simulink model "GS_model"  (R2018b)
settings: Solver=ode5  StartTime=0.0  StopTime=SimuStopTime  FixedStep=T_Simu  RelTol=1e-3
InitFcn:
  | Initial
undefined symbols (not defined in the file or in its folder): Aba10, Aba20, aeroCIP2006_S, aeroCIP2006_X, aeroCIP2006_Y, Agl0, Ass_kS, Ass_n1, Ass_n2, Ass_n3, Ass_n4, Ass_Noise, Ass_R, Ass_Resolution, Ass_TmOrder, AssA_Fix_Abs, AssB_Fix_Abs, AssC_Fix_Abs, AssD_Fix_Abs, AssE_Fix_Aps, AssF_Fix_Aps, C, c_max, c_min, Cd, CenterOfFigNX, CenterOfFigNY, CenterOfFigNZ, CenterOfFigP1, CenterOfFigP2, CenterOfFigPX, CenterOfFigPY, CenterOfFigPZ, Cmu, Crou, DEG2RAD, DiscIntNeverNeededParam, Eg_Dir, Eg_F, Eg_PrepareTime, Eg_r_L_L, Fw_Abf, Fw_Hmax, Fw_J, Fw_Spd0, Fw_Tmax, git_hash_BaseLine, git_hash_Project, Gnss_Noise_Pos, Gnss_Noise_Vel, Gnss_PropgationTime, GyroA_Fix_Abg, GyroA_Noise, GyroB_Fix_Abg, GyroB_Noise, GyroC_Fix_Abg, GyroC_Noise, GyroD_Fix_Abg, GyroD_Noise, h ... (+94)
libraries: simulink x308, sharedutil x46, aerolibutil x37, sharedtransform x31, vrlib x14, aerolibgravity2 x2
(part 5 of 20)

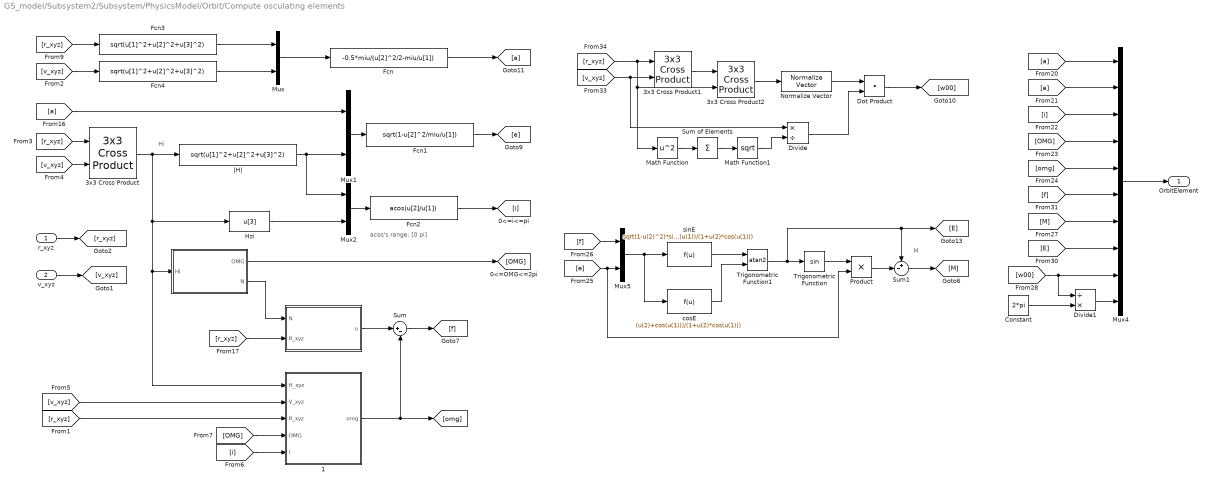
== system GS_model/Subsystem2/Subsystem/PhysicsModel/Orbit/Compute osculating elements ==
  note: Hi
  note: acos's range: [0 pi]
  note: M
  r_xyz : Inport
  v_xyz : Inport  Port=2
  " " : Subsystem
  "     " : Subsystem
  "   1" : Subsystem
  3x3 Cross Product : sharedutil/3x3 Cross Product  aMode=aMode
      settings: SourceProductBaseCode=AE,PW,MT,VE,VP
  3x3 Cross Product1 : sharedutil/3x3 Cross Product  aMode=aMode
      settings: SourceProductBaseCode=AE,PW,MT,VE,VP
  3x3 Cross Product2 : sharedutil/3x3 Cross Product  aMode=aMode
      settings: SourceProductBaseCode=AE,PW,MT,VE,VP
  Constant : Constant  Value=2*pi
  Divide : Product  Inputs=*/
  Divide1 : Product  Inputs=/*
  Dot Product : DotProduct  InputSameDT=on  OutDataTypeStr=Inherit: Inherit via internal rule
  Fcn : Fcn  Expr=-0.5*miu/(u[2]^2/2-miu/u[1])
  Fcn1 : Fcn  Expr=sqrt(1-u[2]^2/miu/u[1])
  Fcn2 : Fcn  Expr=acos(u[2]/u[1])
  Fcn3 : Fcn  Expr=sqrt(u[1]^2+u[2]^2+u[3]^2)
  Fcn4 : Fcn  Expr=sqrt(u[1]^2+u[2]^2+u[3]^2)
  Hzi : Fcn  Expr=u[3]
  Math Function : Math  Operator=square  SaturateOnIntegerOverflow=on
  Math Function1 : Math  Operator=sqrt  SaturateOnIntegerOverflow=on
  Mux{,1..2,5} (4 alike) : Mux  Inputs=2
  Mux4 : Mux  Inputs=10
  Normalize Vector : vrlib/Utilities/Normalize Vector  maxzero=0
  Product : Product  RndMeth=Zero
  Sum : Sum  Inputs=|+-
  Sum of Elements : Sum  Inputs=+
  Sum1 : Sum  Inputs=+-|
  Trigonometric Function : Trigonometry
  Trigonometric Function1 : Trigonometry  Operator=atan2
  cosE : Fcn  Expr=(u(2)+cos(u(1)))/(1+u(2)*cos(u(1)))
  sinE : Fcn  Expr=sqrt(1-u(2)^2)*sin(u(1))/(1+u(2)*cos(u(1)))
  |H| : Fcn  Expr=sqrt(u[1]^2+u[2]^2+u[3]^2)
  OrbitElement : Outport
  wires:
  [r_xyz] -> Fcn3/1
  [v_xyz] -> Fcn4/1
  Fcn4/1 -> Mux/2
  Mux/1 -> Fcn/1
  Fcn/1 -> [a]
  3x3 Cross Product/1 -> |H|/1, "   1"/1(H_xyz), " "/1(Hi), Hzi/1
  Mux1/1 -> Fcn1/1
  Mux2/1 -> Fcn2/1
  r_xyz/1 -> [r_xyz]
  v_xyz/1 -> [v_xyz]
  [r_xyz] -> "   1"/3(R_xyz)
  [r_xyz] -> 3x3 Cross Product/1
  [v_xyz] -> 3x3 Cross Product/2
  [v_xyz] -> "   1"/2(V_xyz)
  Fcn3/1 -> Mux/1
  |H|/1 -> Mux1/2, Mux2/1
  " "/1(OMG) -> [OMG]
  Fcn1/1 -> [e]
  Fcn2/1 -> [i]
  [a] -> Mux1/1
  "   1"/1(omg) -> Sum/2, [omg]
  Hzi/1 -> Mux2/2
  "     "/1(u) -> Sum/1
  [r_xyz] -> "     "/2(R_xyz)
  Sum/1 -> [f]
  [f] -> Mux5/1
  [e] -> Mux5/2, Product/2
  Mux5/1 -> sinE/1, cosE/1
  Trigonometric Function/1 -> Product/1
  Product/1 -> Sum1/2
  Sum1/1 -> [M]
  Dot Product/1 -> [w00]
  Mux4/1 -> OrbitElement/1
  sinE/1 -> Trigonometric Function1/1
  cosE/1 -> Trigonometric Function1/2
  Trigonometric Function1/1 -> Sum1/1, [E], Trigonometric Function/1
  [r_xyz] -> 3x3 Cross Product1/1, 3x3 Cross Product2/2, Math Function/1
  [v_xyz] -> 3x3 Cross Product1/2, Divide/1
  3x3 Cross Product1/1 -> 3x3 Cross Product2/1
  3x3 Cross Product2/1 -> Normalize Vector/1
  Normalize Vector/1 -> Dot Product/1
  Sum of Elements/1 -> Math Function1/1
  Math Function/1 -> Sum of Elements/1
  Math Function1/1 -> Divide/2
  Divide/1 -> Dot Product/2
  [a] -> Mux4/1
  [e] -> Mux4/2
  [i] -> Mux4/3
  [OMG] -> Mux4/4
  [omg] -> Mux4/5
  [f] -> Mux4/6
  [M] -> Mux4/7
  [E] -> Mux4/8
  [w00] -> Divide1/1, Mux4/9
  Divide1/1 -> Mux4/10
  Constant/1 -> Divide1/2
  " "/2(N) -> "     "/1(N)
  [i] -> "   1"/5(i)
  [OMG] -> "   1"/4(OMG)

== system GS_model/Subsystem2/Subsystem/PhysicsModel/Orbit/Engine ==
  F_Engine(b) : Inport
  Qib : Inport  Port=2
  Math Function : Math  Operator=transpose  SaturateOnIntegerOverflow=on
  Product2 : Product  Multiplication=Matrix(*)
  Quaternions to Direction Cosine Matrix1 : sharedtransform/Quaternions to  Direction Cosine Matrix  aMode=aMode
      settings: SourceProductBaseCode=AE,PW,MT,VE,VP
  F_Engine(i) : Outport
  wires:
  F_Engine(b)/1 -> Product2/2
  Math Function/1 -> Product2/1
  Product2/1 -> F_Engine(i)/1
  Qib/1 -> Quaternions to Direction Cosine Matrix1/1
  Quaternions to Direction Cosine Matrix1/1 -> Math Function/1

== system GS_model/Subsystem2/Subsystem/PhysicsModel/Orbit/Qob 2 Qib ==
  note: u
  note: i
  note: OMG
  OrbitElement : Inport
  Fcn : Fcn  Expr=u(4)
  Fcn1 : Fcn  Expr=u(3)
  Fcn2 : Fcn  Expr=u(5)+u(6)
  Mux : Mux  Inputs=3
  Quaternion Multiplication : aerolibutil/Quaternion Multiplication
  Rotation Angles to Quaternions : sharedtransform/Rotation Angles to Quaternions  rotationOrder=ZXZ  aMode=aMode
      settings: SourceProductBaseCode=AE,PW,MT,VE,VP
  qpo : Constant  Value=[0.5 -0.5 -0.5 0.5]
  Qio : Outport
  wires:
  Rotation Angles to Quaternions/1 -> Quaternion Multiplication/1
  qpo/1 -> Quaternion Multiplication/2
  Quaternion Multiplication/1 -> Qio/1
  OrbitElement/1 -> Fcn2/1, Fcn/1, Fcn1/1
  Fcn1/1 -> Mux/2
  Fcn/1 -> Mux/1
  Fcn2/1 -> Mux/3
  Mux/1 -> Rotation Angles to Quaternions/1

== system GS_model/Subsystem2/Subsystem/PhysicsModel/Orbit/RV_i2RV_f ==
  R_i : Inport
  V_i : Inport  Port=2
  Afi : Inport  Port=3
  Constant : Constant  Value=[0;0;we]
  Cross Product : vrlib/Utilities/Cross Product
  MatrixMultiply : Product  Multiplication=Matrix(*)
  MatrixMultiply1 : Product  Multiplication=Matrix(*)
  Sum : Sum  Inputs=-+|
  R_f : Outport
  V_f : Outport  Port=2
  wires:
  MatrixMultiply/1 -> Cross Product/2, R_f/1
  Afi/1 -> MatrixMultiply/1, MatrixMultiply1/1
  R_i/1 -> MatrixMultiply/2
  V_i/1 -> MatrixMultiply1/2
  MatrixMultiply1/1 -> Sum/2
  Constant/1 -> Cross Product/1
  Cross Product/1 -> Sum/1
  Sum/1 -> V_f/1

== system GS_model/Subsystem2/Subsystem/PhysicsModel/Orbit/Subsystem ==
  Tc_Orbit_Reset : Inport
  RV0 : Inport  Port=2
  a_Perturbation : Inport  Port=3
  F_EP : Inport  Port=4
  Demux : Demux  Outputs=[3;3]
  Gain : Gain  Gain=1/m
  Integrator : Integrator  ExternalReset=level  InitialConditionSource=external
  Integrator1 : Integrator  ExternalReset=level  InitialConditionSource=external
  Sum : Sum  Inputs=|++
  R_i : Outport
  V_i : Outport  Port=2
  wires:
  Integrator/1 -> Integrator1/1, V_i/1
  Tc_Orbit_Reset/1 -> Integrator1/2, Integrator/2
  F_EP/1 -> Gain/1
  Sum/1 -> Integrator/1
  a_Perturbation/1 -> Sum/1
  Demux/1 -> Integrator1/3
  Demux/2 -> Integrator/3
  Integrator1/1 -> R_i/1
  RV0/1 -> Demux/1
  Gain/1 -> Sum/2

== system GS_model/Subsystem2/Subsystem/PhysicsModel/Orbit/Subsystem1 ==
  UTC_1970 : Inport
  Constant : Constant  Value=aeroCIP2006_X
  Constant1 : Constant  Value=aeroCIP2006_Y
  Constant3 : Constant  Value=aeroCIP2006_S
  DcmECI2ECEF : MATLAB Function  TreatAsAtomicUnit=on
  Demux : Demux  Outputs=14
  From File : FromFile  FileName=EOP_data_in.mat  OutDataTypeStr=double  SampleTime=0
  Gain{3..6} (4 alike) : Gain  Gain=1/3600/180*pi
  Mux : Mux  Inputs=2
  Mux1 : Mux  Inputs=2
  Terminator{,1..7} (8 alike) : Terminator
  Afi : Outport
  wires:
  Demux/7 -> Gain4/1
  Demux/9 -> Terminator4/1
  From File/1 -> Demux/1
  Demux/14 -> DcmECI2ECEF/7(deltaAT)
  Demux/13 -> Gain6/1
  Gain6/1 -> Mux1/2
  Demux/11 -> Terminator6/1
  Mux1/1 -> DcmECI2ECEF/6(dCIP)
  Demux/6 -> Gain3/1
  Demux/4 -> Terminator2/1
  Demux/3 -> Terminator1/1
  Demux/8 -> DcmECI2ECEF/5(deltaUT1)
  Gain5/1 -> Mux1/1
  Demux/5 -> Terminator3/1
  Demux/12 -> Gain5/1
  Mux/1 -> DcmECI2ECEF/4(polarMotion)
  Gain3/1 -> Mux/1
  Gain4/1 -> Mux/2
  Demux/10 -> Terminator5/1
  Demux/2 -> Terminator/1
  Demux/1 -> Terminator7/1
  UTC_1970/1 -> DcmECI2ECEF/8(Seconds)
  DcmECI2ECEF/1(y) -> Afi/1
  Constant/1 -> DcmECI2ECEF/2(aeroCIP2006_X)
  Constant1/1 -> DcmECI2ECEF/1(aeroCIP2006_Y)
  Constant3/1 -> DcmECI2ECEF/3(aeroCIP2006_S)

== system GS_model/Subsystem2/Subsystem/PhysicsModel/Subsystem3/Subsystem1 ==
  note: A_a0a
  note: A_p0p
  Agl/w/a_SADA : Inport
  Constant : Constant  Value=round(SADA_RotateOrder/100)
  Constant1 : Constant  Value=Aba10
  Constant2 : Constant  Value=Aba20
  Constant3 : Constant  Value=round(mod(SADA_RotateOrder,100)/10)
  MATLAB Function : MATLAB Function  TreatAsAtomicUnit=on
  MATLAB Function1 : MATLAB Function  TreatAsAtomicUnit=on
  MATLAB Function2 : MATLAB Function  TreatAsAtomicUnit=on
  MATLAB Function3 : MATLAB Function  TreatAsAtomicUnit=on
  Product{1..4} (4 alike) : Product  Multiplication=Matrix(*)  SaturateOnIntegerOverflow=on  InputSameDT=on  OutDataTypeStr=Inherit: Same as first input
  Selector : Selector  InputPortWidth=12  IndexOptions=Index vector (dialog)  Indices=[1]  OutputSizes=1
  Selector1 : Selector  InputPortWidth=12  IndexOptions=Index vector (dialog)  Indices=7  OutputSizes=1
  Selector4 : Selector  InputPortWidth=12  IndexOptions=Index vector (dialog)  Indices=4  OutputSizes=1
  Selector5 : Selector  InputPortWidth=12  IndexOptions=Index vector (dialog)  Indices=10  OutputSizes=1
  Transpose{,1..3} (4 alike) : Math  Operator=transpose  SaturateOnIntegerOverflow=on
  Abp1 : Outport
  Aba1 : Outport  Port=2
  Abp2 : Outport  Port=3
  Aba2 : Outport  Port=4
  wires:
  Transpose/1 -> Product2/2
  Transpose3/1 -> Product4/2
  Selector/1 -> MATLAB Function/1(Agl)
  Transpose2/1 -> Product3/2
  MATLAB Function3/1(A) -> Transpose3/1
  MATLAB Function/1(A) -> Transpose/1
  Transpose1/1 -> Product1/2
  Constant1/1 -> Product2/1
  Agl/w/a_SADA/1 -> Selector/1, Selector5/1, Selector1/1, Selector4/1
  Constant2/1 -> Product3/1
  MATLAB Function2/1(A) -> Transpose2/1
  MATLAB Function1/1(A) -> Transpose1/1
  Constant/1 -> MATLAB Function2/2(Order), MATLAB Function/2(Order)
  Selector4/1 -> MATLAB Function1/1(Agl)
  Constant3/1 -> MATLAB Function1/2(Order), MATLAB Function3/2(Order)
  Selector1/1 -> MATLAB Function2/1(Agl)
  Selector5/1 -> MATLAB Function3/1(Agl)
  Product2/1 -> Product1/1, Aba1/1
  Product1/1 -> Abp1/1
  Product3/1 -> Product4/1, Aba2/1
  Product4/1 -> Abp2/1

== system GS_model/Subsystem2/Subsystem/PhysicsModel/Time/Subsystem ==
  In1 : Inport
  Trigger : TriggerPort  TriggerType=falling  VariantControl=Variant  PortDimensions=1
  Out1 : Outport
  wires:
  In1/1 -> Out1/1

== system GS_model/Subsystem2/Subsystem/Sensor/Ass/BodyAss(A&B&C&D)Model ==
  Sunshine : Inport
  Sun_b : Inport  Port=2
  TC_Ass : Inport  Port=3
  Constant : Constant  Value=AssA_Fix_Abs
  Constant1 : Constant  Value=Ass_kS
  Constant2 : Constant
  Constant3 : Constant  Value=AssB_Fix_Abs
  Constant4 : Constant  Value=AssC_Fix_Abs
  Constant5 : Constant  Value=AssD_Fix_Abs
  Constant6 : Constant  Value=2
  Constant7 : Constant  Value=3
  Constant8 : Constant  Value=4
  Mux : Mux
  Subsystem : Subsystem
      mask Display: disp('AssAModel')
  Subsystem1 : Subsystem
      mask Display: disp('AssAModel')
  Subsystem2 : Subsystem
      mask Display: disp('AssAModel')
  Subsystem3 : Subsystem
      mask Display: disp('AssAModel')
  TM_Data_AssA&B&C&D : Outport
  wires:
  Subsystem3/1(TM_Data_AssA) -> Mux/4
  Sun_b/1 -> Subsystem1/3(Sun_b), Subsystem3/3(Sun_b), Subsystem2/3(Sun_b), Subsystem/3(Sun_b)
  Sunshine/1 -> Subsystem1/1(Sunshine), Subsystem3/1(Sunshine), Subsystem2/1(Sunshine), Subsystem/1(Sunshine)
  Subsystem1/1(TM_Data_AssA) -> Mux/2
  Constant1/1 -> Subsystem1/4(kS_Ass), Subsystem3/4(kS_Ass), Subsystem2/4(kS_Ass), Subsystem/4(kS_Ass)
  Constant5/1 -> Subsystem3/2(AbAss)
  TC_Ass/1 -> Subsystem1/5(TC_Ass), Subsystem3/5(TC_Ass), Subsystem2/5(TC_Ass), Subsystem/5(TC_Ass)
  Constant/1 -> Subsystem/2(AbAss)
  Constant3/1 -> Subsystem1/2(AbAss)
  Constant4/1 -> Subsystem2/2(AbAss)
  Subsystem/1(TM_Data_AssA) -> Mux/1
  Subsystem2/1(TM_Data_AssA) -> Mux/3
  Mux/1 -> TM_Data_AssA&B&C&D/1
  Constant2/1 -> Subsystem/6(AssNum)
  Constant6/1 -> Subsystem1/6(AssNum)
  Constant7/1 -> Subsystem2/6(AssNum)
  Constant8/1 -> Subsystem3/6(AssNum)

== system GS_model/Subsystem2/Subsystem/Sensor/Ass/SolarPanelAss(E&F)Model ==
  Sunshine : Inport
  Sun_b : Inport  Port=2
  TC_Ass : Inport  Port=3
  Abp_PY : Inport  Port=4
  Abp_NY : Inport  Port=5
  Constant : Constant  Value=AssE_Fix_Aps
  Constant1 : Constant  Value=Ass_kS
  Constant2 : Constant  Value=5
  Constant3 : Constant  Value=AssF_Fix_Aps
  Constant4 : Constant  Value=6
  Mux : Mux  Inputs=2
  Subsystem : Subsystem
      mask Display: disp('AssEModel')
  Subsystem1 : Subsystem
      mask Display: disp('AssFModel')
  TM_Data_AssE&F : Outport
  wires:
  Mux/1 -> TM_Data_AssE&F/1
  Subsystem/1(TM_Data_AssE) -> Mux/1
  Constant3/1 -> Subsystem1/2(ApAss)
  Constant/1 -> Subsystem/2(ApAss)
  Constant1/1 -> Subsystem1/4(kS_Ass), Subsystem/4(kS_Ass)
  Subsystem1/1(TM_Data_AssF) -> Mux/2
  Sunshine/1 -> Subsystem1/1(Sunshine), Subsystem/1(Sunshine)
  Sun_b/1 -> Subsystem1/3(Sun_b), Subsystem/3(Sun_b)
  Abp_PY/1 -> Subsystem/6(Abp_PY)
  TC_Ass/1 -> Subsystem1/5(TC_Ass), Subsystem/5(TC_Ass)
  Abp_NY/1 -> Subsystem1/6(Abp_NY)
  Constant2/1 -> Subsystem/7(AssNum)
  Constant4/1 -> Subsystem1/7(AssNum)

== system GS_model/Subsystem2/Subsystem/Sensor/GNSS/Enabled Subsystem ==
  In1 : Inport
  Trigger : TriggerPort  VariantControl=Variant  PortDimensions=1
  Out1 : Outport
  wires:
  In1/1 -> Out1/1

== system GS_model/Subsystem2/Subsystem/Sensor/GNSS/GNSSErrModel ==
  note: TC_GNSS_GNDSet_Pos[4*1]
  note: TC_GNSSErr_Pos_Constant[2*1]
  note: TC_GNSSErr_Spd_Constant[2*1]
  note: TC_GNSSErr_Pos_WildValue[1*1]
  note: TC_GNSSErr_Spd_WildValue[1*1]
  note: TC_GNSS_GNDSet_Spd[4*1]
  note: TC_GNSS_PropagationTime[1*1]
  TC_GNSS : Inport
  R_84 : Inport  Port=2
  V_84 : Inport  Port=3
  Demux : Demux  Outputs=[4;2;1;4;2;1;2]
  GNSSErrSet_Pos : Subsystem
      mask Display: disp('GNSSErrSet_Constant')
  GNSSErrSet_Pos1 : Subsystem
      mask Display: disp('GNSSErrSet_WildValue')
  TM_R_84 : Outport
  TM_V_84 : Outport  Port=2
  TC_GNSS_PropagationTime : Outport  Port=3
  wires:
  TC_GNSS/1 -> Demux/1
  Demux/6 -> GNSSErrSet_Pos1/3(TC_GNSSErr_Spd_WildValue)
  Demux/5 -> GNSSErrSet_Pos1/2(TC_GNSSErr_Spd_Constant)
  Demux/3 -> GNSSErrSet_Pos/4(TC_GNSSErr_Pos_WildValue)
  Demux/1 -> GNSSErrSet_Pos/2(TC_GNSS_GNDSet_Pos)
  Demux/2 -> GNSSErrSet_Pos/3(TC_GNSSErr_Pos_Constant)
  R_84/1 -> GNSSErrSet_Pos/1(R_84)
  Demux/4 -> GNSSErrSet_Pos1/1(TC_GNSS_GNDSet_Spd)
  V_84/1 -> GNSSErrSet_Pos1/4(V_84)
  GNSSErrSet_Pos/1(TM_R_84) -> TM_R_84/1
  GNSSErrSet_Pos1/1(TM_V_84) -> TM_V_84/1
  Demux/7 -> TC_GNSS_PropagationTime/1

== system GS_model/Subsystem2/Subsystem/Sensor/GNSS/GNSS_IntegerSecond_Judge ==
  TAI1970 : Inport
  Compare To Constant : simulink/Logic and Bit Operations/Compare To Constant  relop=<=  const=T_Simu/2  OutDataTypeStr=boolean
  Compare To Constant1 : simulink/Logic and Bit Operations/Compare To Constant  relop=<  const=T_Simu/2  OutDataTypeStr=boolean
  Constant : Constant
  Logical Operator : Logic  Operator=OR  AllPortsSameDT=off  OutDataTypeStr=boolean
  Math Function : Math  Operator=mod  SaturateOnIntegerOverflow=on
  Sum : Sum  Inputs=|+-
  Boolean : Outport
  wires:
  Sum/1 -> Compare To Constant1/1
  Math Function/1 -> Sum/2, Compare To Constant/1
  Constant/1 -> Math Function/2, Sum/1
  Compare To Constant1/1 -> Logical Operator/1
  Compare To Constant/1 -> Logical Operator/2
  TAI1970/1 -> Math Function/1
  Logical Operator/1 -> Boolean/1

== system GS_model/Subsystem2/Subsystem/Sensor/GNSS/Orbit ==
  note: a
  note: e
  note: i
  note: OMG
  note: omg
  note: M
  note: E
  note: w00
  note: w00/2pi
  note: f0+T*w0
  "\tTC_GNSS_PropagationTime" : Inport
  UTC_1970 : Inport  Port=2
  Demux : Demux  Outputs=2
  Demux1 : Demux  Outputs=10
  Dot Product1 : DotProduct  InputSameDT=on  OutDataTypeStr=Inherit: Inherit via internal rule
  MATLAB Function2 : MATLAB Function  TreatAsAtomicUnit=on
  Mux4 : Mux  Inputs=10
  RV_i2RV_f1 : Subsystem
  Subsystem1 : Subsystem
  Sum : Sum  Inputs=|++
  Sum1 : Sum  Inputs=|++
  R_f : Outport
  V_f : Outport  Port=2
  wires:
  Mux4/1 -> MATLAB Function2/1(Orbit)
  Subsystem1/1(Afi) -> RV_i2RV_f1/3(Afi)
  MATLAB Function2/1(RV_i) -> Demux/1
  Demux/1 -> RV_i2RV_f1/1(R_i)
  Demux/2 -> RV_i2RV_f1/2(V_i)
  RV_i2RV_f1/1(R_f) -> R_f/1
  RV_i2RV_f1/2(V_f) -> V_f/1
  [Orbit] -> Demux1/1
  Demux1/1 -> Mux4/1
  Demux1/2 -> Mux4/2
  Demux1/3 -> Mux4/3
  Demux1/4 -> Mux4/4
  Demux1/5 -> Mux4/5
  Demux1/7 -> Mux4/7
  Demux1/8 -> Mux4/8
  Demux1/9 -> Mux4/9, Dot Product1/1
  Demux1/10 -> Mux4/10
  Sum/1 -> Mux4/6
  "\tTC_GNSS_PropagationTime"/1 -> Sum1/2, Dot Product1/2
  Dot Product1/1 -> Sum/2
  Demux1/6 -> Sum/1
  UTC_1970/1 -> Sum1/1
  Sum1/1 -> Subsystem1/1(UTC_1970)

== system GS_model/Subsystem2/Subsystem/Sensor/GNSS/Orbit1 ==
  note: f0+T*w0
  note: w00/2pi
  note: w00
  note: E
  note: M
  note: omg
  note: OMG
  note: i
  note: e
  note: a
  "\tTC_GNSS_PropagationTime" : Inport
  UTC_1970 : Inport  Port=2
  Demux : Demux  Outputs=2
  Demux1 : Demux  Outputs=10
  Dot Product1 : DotProduct  InputSameDT=on  OutDataTypeStr=Inherit: Inherit via internal rule
  MATLAB Function2 : MATLAB Function  TreatAsAtomicUnit=on
  Mux4 : Mux  Inputs=10
  RV_i2RV_f1 : Subsystem
  Subsystem1 : Subsystem
  Sum : Sum  Inputs=|++
  Sum1 : Sum  Inputs=|++
  R_f : Outport
  V_f : Outport  Port=2
  wires:
  Sum1/1 -> Subsystem1/1(UTC_1970)
  UTC_1970/1 -> Sum1/1
  Demux1/6 -> Sum/1
  Dot Product1/1 -> Sum/2
  "\tTC_GNSS_PropagationTime"/1 -> Dot Product1/2, Sum1/2
  Sum/1 -> Mux4/6
  Demux1/10 -> Mux4/10
  Demux1/9 -> Dot Product1/1, Mux4/9
  Demux1/8 -> Mux4/8
  Demux1/7 -> Mux4/7
  Demux1/5 -> Mux4/5
  Demux1/4 -> Mux4/4
  Demux1/3 -> Mux4/3
  Demux1/2 -> Mux4/2
  Demux1/1 -> Mux4/1
  [Orbit] -> Demux1/1
  RV_i2RV_f1/2(V_f) -> V_f/1
  RV_i2RV_f1/1(R_f) -> R_f/1
  Demux/2 -> RV_i2RV_f1/2(V_i)
  Demux/1 -> RV_i2RV_f1/1(R_i)
  MATLAB Function2/1(RV_i) -> Demux/1
  Subsystem1/1(Afi) -> RV_i2RV_f1/3(Afi)
  Mux4/1 -> MATLAB Function2/1(Orbit)

== system GS_model/Subsystem2/Subsystem/Sensor/Gyro/GyroAModel ==
  Wbi_b : Inport
  Gyro_Fix_Abg : Inport  Port=2
  Gyro_Noise : Inport  Port=3
  TC_Gyro : Inport  Port=4
  Gyro_Num : Inport  Port=5
  Demux : Demux  Outputs=[20;4]
  GyroErrSet : Subsystem
  GyroMathModel : Subsystem
  TM_Gyro_Wgi : Outport
  wires:
  Wbi_b/1 -> GyroMathModel/1(Wbi_b)
  Gyro_Fix_Abg/1 -> GyroMathModel/2(Gyro_Fix_Abg)
  Gyro_Noise/1 -> GyroMathModel/4(Gyro_Noise)
  Gyro_Num/1 -> GyroErrSet/3(Gyro_Num), GyroMathModel/5("Gyro_Num ")
  GyroMathModel/1(Wgi_g) -> GyroErrSet/1(Wgi)
  GyroErrSet/1(TM_Gyro_Wgi) -> TM_Gyro_Wgi/1
  TC_Gyro/1 -> Demux/1
  Demux/1 -> GyroErrSet/2(TC_Gyro)
  Demux/2 -> GyroMathModel/3(Gyro_Drift)

== system GS_model/Subsystem2/Subsystem/Sensor/Gyro/GyroBModel ==
  Wbi_b : Inport
  Gyro_Fix_Abg : Inport  Port=2
  Gyro_Noise : Inport  Port=3
  TC_Gyro : Inport  Port=4
  Gyro_Num : Inport  Port=5
  Demux : Demux  Outputs=[20;4]
  GyroErrSet : Subsystem
  GyroMathModel : Subsystem
  TM_Gyro_Wgi : Outport
  wires:
  Demux/2 -> GyroMathModel/3(Gyro_Drift)
  Demux/1 -> GyroErrSet/2(TC_Gyro)
  TC_Gyro/1 -> Demux/1
  GyroErrSet/1(TM_Gyro_Wgi) -> TM_Gyro_Wgi/1
  GyroMathModel/1(Wgi_g) -> GyroErrSet/1(Wgi)
  Gyro_Num/1 -> GyroErrSet/3(Gyro_Num), GyroMathModel/5("Gyro_Num ")
  Gyro_Noise/1 -> GyroMathModel/4(Gyro_Noise)
  Gyro_Fix_Abg/1 -> GyroMathModel/2(Gyro_Fix_Abg)
  Wbi_b/1 -> GyroMathModel/1(Wbi_b)

== system GS_model/Subsystem2/Subsystem/Sensor/Gyro/GyroCModel ==
  Wbi_b : Inport
  Gyro_Fix_Abg : Inport  Port=2
  Gyro_Noise : Inport  Port=3
  TC_Gyro : Inport  Port=4
  Gyro_Num : Inport  Port=5
  Demux : Demux  Outputs=[20;4]
  GyroErrSet : Subsystem
  GyroMathModel : Subsystem
  TM_Gyro_Wgi : Outport
  wires:
  Wbi_b/1 -> GyroMathModel/1(Wbi_b)
  Gyro_Fix_Abg/1 -> GyroMathModel/2(Gyro_Fix_Abg)
  Gyro_Noise/1 -> GyroMathModel/4(Gyro_Noise)
  Gyro_Num/1 -> GyroErrSet/3(Gyro_Num), GyroMathModel/5("Gyro_Num ")
  GyroMathModel/1(Wgi_g) -> GyroErrSet/1(Wgi)
  GyroErrSet/1(TM_Gyro_Wgi) -> TM_Gyro_Wgi/1
  TC_Gyro/1 -> Demux/1
  Demux/1 -> GyroErrSet/2(TC_Gyro)
  Demux/2 -> GyroMathModel/3(Gyro_Drift)

== system GS_model/Subsystem2/Subsystem/Sensor/Gyro/GyroDModel ==
  Wbi_b : Inport
  Gyro_Fix_Abg : Inport  Port=2
  Gyro_Noise : Inport  Port=3
  TC_Gyro : Inport  Port=4
  Gyro_Num : Inport  Port=5
  Demux : Demux  Outputs=[20;4]
  GyroErrSet : Subsystem
  GyroMathModel : Subsystem
  TM_Gyro_Wgi : Outport
  wires:
  Demux/2 -> GyroMathModel/3(Gyro_Drift)
  Demux/1 -> GyroErrSet/2(TC_Gyro)
  TC_Gyro/1 -> Demux/1
  GyroErrSet/1(TM_Gyro_Wgi) -> TM_Gyro_Wgi/1
  GyroMathModel/1(Wgi_g) -> GyroErrSet/1(Wgi)
  Gyro_Num/1 -> GyroErrSet/3(Gyro_Num), GyroMathModel/5("Gyro_Num ")
  Gyro_Noise/1 -> GyroMathModel/4(Gyro_Noise)
  Gyro_Fix_Abg/1 -> GyroMathModel/2(Gyro_Fix_Abg)
  Wbi_b/1 -> GyroMathModel/1(Wbi_b)

== system GS_model/Subsystem2/Subsystem/Sensor/Magnetometer/MmModel1 ==
  Bb : Inport
  M_Mt : Inport  Port=2
  Mm_Fix_Abm : Inport  Port=3
  Mm_MtInflunce_Coff : Inport  Port=4
  Mm_Noise : Inport  Port=5
  TC_Mm : Inport  Port=6
  Mm_Num : Inport  Port=7
  Mm_ErrSet : Subsystem
  Mm_MathModel : Subsystem
  TM_Mm : Outport
  wires:
  Mm_Fix_Abm/1 -> Mm_MathModel/2(Mm_Fix_Abm)
  Bb/1 -> Mm_MathModel/1(Bb)
  Mm_MtInflunce_Coff/1 -> Mm_MathModel/3(Mm_MtInflunce_Coff)
  Mm_Noise/1 -> Mm_MathModel/4(Mm_Noise)
  Mm_MathModel/1(Mm_MagneticIntensity) -> Mm_ErrSet/1(Mm_MagneticIntensity)
  Mm_ErrSet/1(TM_Mm) -> TM_Mm/1
  TC_Mm/1 -> Mm_ErrSet/3(TC_Mm)
  Mm_Num/1 -> Mm_ErrSet/2(Mm_Num)
  M_Mt/1 -> Mm_MathModel/5(M_Mt)

== system GS_model/Subsystem2/Subsystem/Sensor/Magnetometer/MmModel2 ==
  Bb : Inport
  M_Mt : Inport  Port=2
  Mm_Fix_Abm : Inport  Port=3
  Mm_MtInflunce_Coff : Inport  Port=4
  Mm_Noise : Inport  Port=5
  TC_Mm : Inport  Port=6
  Mm_Num : Inport  Port=7
  Mm_ErrSet : Subsystem
  Mm_MathModel : Subsystem
  TM_Mm : Outport
  wires:
  M_Mt/1 -> Mm_MathModel/5(MtCoff)
  Mm_Num/1 -> Mm_ErrSet/2(Mm_Num)
  TC_Mm/1 -> Mm_ErrSet/3(TC_Mm)
  Mm_ErrSet/1(TM_Mm) -> TM_Mm/1
  Mm_MathModel/1(Mm_MagneticIntensity) -> Mm_ErrSet/1(Mm_MagneticIntensity)
  Mm_Noise/1 -> Mm_MathModel/4(Mm_Noise)
  Mm_MtInflunce_Coff/1 -> Mm_MathModel/3(Mm_MtInflunce_Coff)
  Bb/1 -> Mm_MathModel/1(Bb)
  Mm_Fix_Abm/1 -> Mm_MathModel/2(Mm_Fix_Abm)

== system GS_model/Subsystem2/Subsystem/Sensor/Magnetometer/MmModel3 ==
  Bb : Inport
  M_Mt : Inport  Port=2
  Mm_Fix_Abm : Inport  Port=3
  Mm_MtInflunce_Coff : Inport  Port=4
  Mm_Noise : Inport  Port=5
  TC_Mm : Inport  Port=6
  Mm_Num : Inport  Port=7
  Mm_ErrSet : Subsystem
  Mm_MathModel : Subsystem
  TM_Mm : Outport
  wires:
  Mm_Fix_Abm/1 -> Mm_MathModel/2(Mm_Fix_Abm)
  Bb/1 -> Mm_MathModel/1(Bb)
  Mm_MtInflunce_Coff/1 -> Mm_MathModel/3(Mm_MtInflunce_Coff)
  Mm_Noise/1 -> Mm_MathModel/4(Mm_Noise)
  Mm_MathModel/1(Mm_MagneticIntensity) -> Mm_ErrSet/1(Mm_MagneticIntensity)
  Mm_ErrSet/1(TM_Mm) -> TM_Mm/1
  TC_Mm/1 -> Mm_ErrSet/3(TC_Mm)
  Mm_Num/1 -> Mm_ErrSet/2(Mm_Num)
  M_Mt/1 -> Mm_MathModel/5(MtCoff)

== system GS_model/Subsystem2/Subsystem/Sensor/Magnetometer/MmModel4 ==
  Bb : Inport
  M_Mt : Inport  Port=2
  Mm_Fix_Abm : Inport  Port=3
  Mm_MtInflunce_Coff : Inport  Port=4
  Mm_Noise : Inport  Port=5
  TC_Mm : Inport  Port=6
  Mm_Num : Inport  Port=7
  Mm_ErrSet : Subsystem
  Mm_MathModel : Subsystem
  TM_Mm : Outport
  wires:
  M_Mt/1 -> Mm_MathModel/5(MtCoff)
  Mm_Num/1 -> Mm_ErrSet/2(Mm_Num)
  TC_Mm/1 -> Mm_ErrSet/3(TC_Mm)
  Mm_ErrSet/1(TM_Mm) -> TM_Mm/1
  Mm_MathModel/1(Mm_MagneticIntensity) -> Mm_ErrSet/1(Mm_MagneticIntensity)
  Mm_Noise/1 -> Mm_MathModel/4(Mm_Noise)
  Mm_MtInflunce_Coff/1 -> Mm_MathModel/3(Mm_MtInflunce_Coff)
  Bb/1 -> Mm_MathModel/1(Bb)
  Mm_Fix_Abm/1 -> Mm_MathModel/2(Mm_Fix_Abm)

== system GS_model/Subsystem2/Subsystem/Sensor/StA&B&C&DModel1/StAMathModel ==
  note: TC_StFixErr[5*1]
  note: TC_StNoiseCoff[2*1]
  note: TC_StErr_Constant[2*1]
  note: TC_StErr_WildValue[2*1]
  note: TC_StErr_Jump[4*1]
  note: TC_StErr_Fluctuation[3*1]
  note: TC_StGNDSet[6*1]
  Qib : Inport
  Cons_StNoise : Inport  Port=2
  Qsb_StAFix : Inport  Port=3
  TC_St : Inport  Port=4
  StNum : Inport  Port=5
  Sun_b : Inport  Port=6
  Sunshine : Inport  Port=7
  SEA : Inport  Port=8
  EEA : Inport  Port=9
  Qob : Inport  Port=10
  Demux : Demux  Outputs=[2;5;2;6;2;2;4;3]
  Mux : Mux  Inputs=2
  StErrSet : Subsystem
  StMathModel : Subsystem
  Subsystem : Subsystem
  TM_Data_StA : Outport
  Agl_St&SunEarth : Outport  Port=2
  wires:
  Qib/1 -> StMathModel/1(Qib)
  Qsb_StAFix/1 -> Subsystem/4(Qsb_StAFix), StMathModel/3(Qsb_StFix)
  Demux/2 -> StMathModel/4(TC_StFixErr)
  TC_St/1 -> Demux/1
  Demux/4 -> StErrSet/3(TC_StGNDSet)
  Mux/1 -> TM_Data_StA/1
  Cons_StNoise/1 -> StMathModel/2(Cons_StNoise)
  StNum/1 -> Subsystem/9(StNum), StErrSet/2(StNum), StMathModel/6(StNum)
  Demux/8 -> StErrSet/7(TC_StErr_Fluctuation)
  Demux/7 -> StErrSet/6(TC_StErr_Jump)
  Demux/6 -> StErrSet/5(TC_StErr_WildValue)
  Demux/5 -> StErrSet/4(TC_StErr_Constant)
  Demux/3 -> StMathModel/5(TC_StNoiseCoff)
  StMathModel/1(Qis_St) -> Subsystem/8(Qis)
  Subsystem/3(Qis_St) -> StErrSet/1(Qis_St)
  EEA/1 -> Subsystem/6(EEA)
  SEA/1 -> Subsystem/5(SEA)
  Qob/1 -> Subsystem/7(Qob)
  Sun_b/1 -> Subsystem/1(Sun_b)
  Sunshine/1 -> Subsystem/2(Sunshine)
  Subsystem/1(Agl_St&SunEarth) -> Agl_St&SunEarth/1
  Subsystem/2(Valid) -> Mux/1
  Demux/1 -> Subsystem/3(Tc_ValidSet)
  StErrSet/1(TM_St_Qis/w) -> Mux/2

== system GS_model/Subsystem2/Subsystem/Sensor/StA&B&C&DModel1/StAMathModel1 ==
  note: TC_StGNDSet[6*1]
  note: TC_StErr_Fluctuation[3*1]
  note: TC_StErr_Jump[4*1]
  note: TC_StErr_WildValue[2*1]
  note: TC_StErr_Constant[2*1]
  note: TC_StNoiseCoff[2*1]
  note: TC_StFixErr[5*1]
  Qib : Inport
  Cons_StNoise : Inport  Port=2
  Qsb_StAFix : Inport  Port=3
  TC_St : Inport  Port=4
  StNum : Inport  Port=5
  Sun_b : Inport  Port=6
  Sunshine : Inport  Port=7
  SEA : Inport  Port=8
  EEA : Inport  Port=9
  Qob : Inport  Port=10
  Demux : Demux  Outputs=[2;5;2;6;2;2;4;3]
  Mux : Mux  Inputs=2
  StErrSet : Subsystem
  StMathModel : Subsystem
  Subsystem : Subsystem
  TM_Data_StA : Outport
  Agl_St&SunEarth : Outport  Port=2
  wires:
  StErrSet/1(TM_St_Qis/w) -> Mux/2
  Demux/1 -> Subsystem/3(Tc_ValidSet)
  Subsystem/2(Valid) -> Mux/1
  Subsystem/1(Agl_St&SunEarth) -> Agl_St&SunEarth/1
  Sunshine/1 -> Subsystem/2(Sunshine)
  Sun_b/1 -> Subsystem/1(Sun_b)
  Qob/1 -> Subsystem/7(Qob)
  SEA/1 -> Subsystem/5(SEA)
  EEA/1 -> Subsystem/6(EEA)
  Subsystem/3(Qis_St) -> StErrSet/1(Qis_St)
  StMathModel/1(Qis_St) -> Subsystem/8(Qis)
  Demux/3 -> StMathModel/5(TC_StNoiseCoff)
  Demux/5 -> StErrSet/4(TC_StErr_Constant)
  Demux/6 -> StErrSet/5(TC_StErr_WildValue)
  Demux/7 -> StErrSet/6(TC_StErr_Jump)
  Demux/8 -> StErrSet/7(TC_StErr_Fluctuation)
  StNum/1 -> StMathModel/6(StNum), StErrSet/2(StNum), Subsystem/9(StNum)
  Cons_StNoise/1 -> StMathModel/2(Cons_StNoise)
  Mux/1 -> TM_Data_StA/1
  Demux/4 -> StErrSet/3(TC_StGNDSet)
  TC_St/1 -> Demux/1
  Demux/2 -> StMathModel/4(TC_StFixErr)
  Qsb_StAFix/1 -> StMathModel/3(Qsb_StFix), Subsystem/4(Qsb_StAFix)
  Qib/1 -> StMathModel/1(Qib)

== system GS_model/Subsystem2/Subsystem/Sensor/StA&B&C&DModel1/StAMathModel2 ==
  note: TC_StFixErr[5*1]
  note: TC_StNoiseCoff[2*1]
  note: TC_StErr_Constant[2*1]
  note: TC_StErr_WildValue[2*1]
  note: TC_StErr_Jump[4*1]
  note: TC_StErr_Fluctuation[3*1]
  note: TC_StGNDSet[6*1]
  Qib : Inport
  Cons_StNoise : Inport  Port=2
  Qsb_StAFix : Inport  Port=3
  TC_St : Inport  Port=4
  StNum : Inport  Port=5
  Sun_b : Inport  Port=6
  Sunshine : Inport  Port=7
  SEA : Inport  Port=8
  EEA : Inport  Port=9
  Qob : Inport  Port=10
  Demux : Demux  Outputs=[2;5;2;6;2;2;4;3]
  Mux : Mux  Inputs=2
  StErrSet : Subsystem
  StMathModel : Subsystem
  Subsystem : Subsystem
  TM_Data_StA : Outport
  Agl_St&SunEarth : Outport  Port=2
  wires:
  Qib/1 -> StMathModel/1(Qib)
  Qsb_StAFix/1 -> Subsystem/4(Qsb_StAFix), StMathModel/3(Qsb_StFix)
  Demux/2 -> StMathModel/4(TC_StFixErr)
  TC_St/1 -> Demux/1
  Demux/4 -> StErrSet/3(TC_StGNDSet)
  Mux/1 -> TM_Data_StA/1
  Cons_StNoise/1 -> StMathModel/2(Cons_StNoise)
  StNum/1 -> Subsystem/9(StNum), StErrSet/2(StNum), StMathModel/6(StNum)
  Demux/8 -> StErrSet/7(TC_StErr_Fluctuation)
  Demux/7 -> StErrSet/6(TC_StErr_Jump)
  Demux/6 -> StErrSet/5(TC_StErr_WildValue)
  Demux/5 -> StErrSet/4(TC_StErr_Constant)
  Demux/3 -> StMathModel/5(TC_StNoiseCoff)
  StMathModel/1(Qis_St) -> Subsystem/8(Qis)
  Subsystem/3(Qis_St) -> StErrSet/1(Qis_St)
  EEA/1 -> Subsystem/6(EEA)
  SEA/1 -> Subsystem/5(SEA)
  Qob/1 -> Subsystem/7(Qob)
  Sun_b/1 -> Subsystem/1(Sun_b)
  Sunshine/1 -> Subsystem/2(Sunshine)
  Subsystem/1(Agl_St&SunEarth) -> Agl_St&SunEarth/1
  Subsystem/2(Valid) -> Mux/1
  Demux/1 -> Subsystem/3(Tc_ValidSet)
  StErrSet/1(TM_St_Qis/w) -> Mux/2

== system GS_model/Subsystem2/Subsystem/Sensor/StA&B&C&DModel1/StAMathModel3 ==
  note: TC_StGNDSet[6*1]
  note: TC_StErr_Fluctuation[3*1]
  note: TC_StErr_Jump[4*1]
  note: TC_StErr_WildValue[2*1]
  note: TC_StErr_Constant[2*1]
  note: TC_StNoiseCoff[2*1]
  note: TC_StFixErr[5*1]
  Qib : Inport
  Cons_StNoise : Inport  Port=2
  Qsb_StAFix : Inport  Port=3
  TC_St : Inport  Port=4
  StNum : Inport  Port=5
  Sun_b : Inport  Port=6
  Sunshine : Inport  Port=7
  SEA : Inport  Port=8
  EEA : Inport  Port=9
  Qob : Inport  Port=10
  Demux : Demux  Outputs=[2;5;2;6;2;2;4;3]
  Mux : Mux  Inputs=2
  StErrSet : Subsystem
  StMathModel : Subsystem
  Subsystem : Subsystem
  TM_Data_StA : Outport
  Agl_St&SunEarth : Outport  Port=2
  wires:
  StErrSet/1(TM_St_Qis/w) -> Mux/2
  Demux/1 -> Subsystem/3(Tc_ValidSet)
  Subsystem/2(Valid) -> Mux/1
  Subsystem/1(Agl_St&SunEarth) -> Agl_St&SunEarth/1
  Sunshine/1 -> Subsystem/2(Sunshine)
  Sun_b/1 -> Subsystem/1(Sun_b)
  Qob/1 -> Subsystem/7(Qob)
  SEA/1 -> Subsystem/5(SEA)
  EEA/1 -> Subsystem/6(EEA)
  Subsystem/3(Qis_St) -> StErrSet/1(Qis_St)
  StMathModel/1(Qis_St) -> Subsystem/8(Qis)
  Demux/3 -> StMathModel/5(TC_StNoiseCoff)
  Demux/5 -> StErrSet/4(TC_StErr_Constant)
  Demux/6 -> StErrSet/5(TC_StErr_WildValue)
  Demux/7 -> StErrSet/6(TC_StErr_Jump)
  Demux/8 -> StErrSet/7(TC_StErr_Fluctuation)
  StNum/1 -> StMathModel/6(StNum), StErrSet/2(StNum), Subsystem/9(StNum)
  Cons_StNoise/1 -> StMathModel/2(Cons_StNoise)
  Mux/1 -> TM_Data_StA/1
  Demux/4 -> StErrSet/3(TC_StGNDSet)
  TC_St/1 -> Demux/1
  Demux/2 -> StMathModel/4(TC_StFixErr)
  Qsb_StAFix/1 -> StMathModel/3(Qsb_StFix), Subsystem/4(Qsb_StAFix)
  Qib/1 -> StMathModel/1(Qib)

== system GS_model/Subsystem2/Subsystem/Sensor/StA&B&C&DModel1/Subsystem ==
  note: St_Second
  note: St_MicroSecond
  UTC_1970 : Inport
  Add3 : Sum  Inputs=-+
  Constant : Constant  Value=St_TimeStamp_leap
  Gain1 : Gain  Gain=1e06  SaturateOnIntegerOverflow=on  OutDataTypeStr=Inherit: Same as input  ParamDataTypeStr=Inherit: Same as input
  Mux : Mux  Inputs=2
  Rounding Function1 : Rounding
  Rounding Function2 : Rounding
  Sum : Sum  Inputs=|++
  St_Time : Outport
  wires:
  Rounding Function1/1 -> Add3/1, Mux/1
  Gain1/1 -> Rounding Function2/1
  Add3/1 -> Gain1/1
  Rounding Function2/1 -> Mux/2
  Mux/1 -> St_Time/1
  UTC_1970/1 -> Sum/1
  Constant/1 -> Sum/2
  Sum/1 -> Add3/2, Rounding Function1/1

== system GS_model/Subsystem2/Tc/Time1/YMDHMS 2 S/Subsystem1 ==
  note: Y
  note: M
  note: D
  note: 3
  note: 1
  note: 2
  In : Inport
  Add : Sum  Inputs=+++--
  Constant1 : Constant  Value=0.5
  Fcn1 : Fcn  Expr=(u(1)-14)/12
  Fcn2 : Fcn  Expr=1461*(u(1)+4800+u(2))/4
  Fcn3 : Fcn  Expr=367*(u(1)-2-u(2)*12)/12
  Fcn4 : Fcn  Expr=(u(1)+4900+u(2))/100
  Fcn5 : Fcn  Expr=3*u(1)/4
  Fcn6 : Fcn  Expr=u(1)-32075
  Mux : Mux  Inputs=2
  Mux1 : Mux  Inputs=2
  Rounding Function{1..5} (5 alike) : Rounding  Operator=fix
  Selector : Selector  InputPortWidth=3  IndexOptions=Index vector (dialog)  Indices=[1]  OutputSizes=1
  Selector1 : Selector  InputPortWidth=3  IndexOptions=Index vector (dialog)  Indices=[2]  OutputSizes=1
  Selector2 : Selector  InputPortWidth=3  IndexOptions=Index vector (dialog)  Indices=[3]  OutputSizes=1
  Out : Outport
  wires:
  Add/1 -> Out/1
  In/1 -> Selector/1, Selector1/1, Selector2/1
  Selector1/1 -> Fcn1/1, Mux1/1
  Fcn1/1 -> Rounding Function1/1
  Rounding Function1/1 -> Mux/2, Mux1/2
  Selector/1 -> Mux/1
  Mux/1 -> Fcn2/1, Fcn4/1
  Fcn2/1 -> Rounding Function2/1
  Mux1/1 -> Fcn3/1
  Fcn3/1 -> Rounding Function3/1
  Fcn4/1 -> Rounding Function4/1
  Rounding Function4/1 -> Fcn5/1
  Fcn5/1 -> Rounding Function5/1
  Selector2/1 -> Fcn6/1
  Fcn6/1 -> Add/1
  Rounding Function2/1 -> Add/2
  Rounding Function3/1 -> Add/3
  Rounding Function5/1 -> Add/4
  Constant1/1 -> Add/5

== system GS_model/Subsystem2/EquipmentCmd/Fw1/Subsystem7/Subsystem1/FWDataSourceChoice ==
  note: 1 -- FW_Spd_422
      | 2 -- FW_Spd_UDP
      | 3 -- FW_Spd_FC
      |
      | 4 -- FW_T_422
      | 5 -- FW_T_UDP
      | 6 -- FW_T_FC
      |
      | 7 -- FW_Mode_422
      | 8 -- FW_Mode_UDP
      | 9 -- FW_Mode_FC
  FW_Data_Source : Inport
  FW_Cmd : Inport  Port=2
  CmdModeChoice : Subsystem
  CmdSpdChoice : Subsystem
  CmdTChoice : Subsystem
  Demux : Demux  Outputs=[3;3;3]
  Cmd_Mode : Outport
  Cmd_Spd : Outport  Port=2
  Cmd_T : Outport  Port=3
  wires:
  FW_Cmd/1 -> Demux/1
  Demux/1 -> CmdSpdChoice/2(FW_CmdSpd)
  Demux/2 -> CmdTChoice/2(FW_CmdTorque)
  CmdTChoice/1(FW_Cmd_T) -> Cmd_T/1
  CmdSpdChoice/1(FW_Cmd_Spd) -> Cmd_Spd/1
  FW_Data_Source/1 -> CmdSpdChoice/1(FW_Data_Source), CmdTChoice/1(FW_Data_Source), CmdModeChoice/1(FW_Data_Source)
  Demux/3 -> CmdModeChoice/2(FW_CmdMode)
  CmdModeChoice/1(FW_Cmd_Mode) -> Cmd_Mode/1

== system GS_model/Subsystem2/EquipmentCmd/Fw1/Subsystem7/Subsystem1/Triggered Subsystem1 ==
  In1 : Inport
  Enable : EnablePort
  Out1 : Outport  InitialOutput=0
  wires:
  In1/1 -> Out1/1

== system GS_model/Subsystem2/EquipmentCmd/Fw1/Subsystem7/Subsystem2/FWDataSourceChoice ==
  note: 1 -- FW_Spd_422
      | 2 -- FW_Spd_UDP
      | 3 -- FW_Spd_FC
      |
      | 4 -- FW_T_422
      | 5 -- FW_T_UDP
      | 6 -- FW_T_FC
      |
      | 7 -- FW_Mode_422
      | 8 -- FW_Mode_UDP
      | 9 -- FW_Mode_FC
  FW_Data_Source : Inport
  FW_Cmd : Inport  Port=2
  CmdModeChoice : Subsystem
  CmdSpdChoice : Subsystem
  CmdTChoice : Subsystem
  Demux : Demux  Outputs=[3;3;3]
  Cmd_Mode : Outport
  Cmd_Spd : Outport  Port=2
  Cmd_T : Outport  Port=3
  wires:
  CmdModeChoice/1(FW_Cmd_Mode) -> Cmd_Mode/1
  Demux/3 -> CmdModeChoice/2(FW_CmdMode)
  FW_Data_Source/1 -> CmdModeChoice/1(FW_Data_Source), CmdTChoice/1(FW_Data_Source), CmdSpdChoice/1(FW_Data_Source)
  CmdSpdChoice/1(FW_Cmd_Spd) -> Cmd_Spd/1
  CmdTChoice/1(FW_Cmd_T) -> Cmd_T/1
  Demux/2 -> CmdTChoice/2(FW_CmdTorque)
  Demux/1 -> CmdSpdChoice/2(FW_CmdSpd)
  FW_Cmd/1 -> Demux/1

== system GS_model/Subsystem2/EquipmentCmd/Fw1/Subsystem7/Subsystem2/Triggered Subsystem1 ==
  In1 : Inport
  Enable : EnablePort
  Out1 : Outport  InitialOutput=0
  wires:
  In1/1 -> Out1/1

== system GS_model/Subsystem2/EquipmentCmd/Fw1/Subsystem7/Subsystem3/FWDataSourceChoice ==
  note: 1 -- FW_Spd_422
      | 2 -- FW_Spd_UDP
      | 3 -- FW_Spd_FC
      |
      | 4 -- FW_T_422
      | 5 -- FW_T_UDP
      | 6 -- FW_T_FC
      |
      | 7 -- FW_Mode_422
      | 8 -- FW_Mode_UDP
      | 9 -- FW_Mode_FC
  FW_Data_Source : Inport
  FW_Cmd : Inport  Port=2
  CmdModeChoice : Subsystem
  CmdSpdChoice : Subsystem
  CmdTChoice : Subsystem
  Demux : Demux  Outputs=[3;3;3]
  Cmd_Mode : Outport
  Cmd_Spd : Outport  Port=2
  Cmd_T : Outport  Port=3
  wires:
  FW_Cmd/1 -> Demux/1
  Demux/1 -> CmdSpdChoice/2(FW_CmdSpd)
  Demux/2 -> CmdTChoice/2(FW_CmdTorque)
  CmdTChoice/1(FW_Cmd_T) -> Cmd_T/1
  CmdSpdChoice/1(FW_Cmd_Spd) -> Cmd_Spd/1
  FW_Data_Source/1 -> CmdSpdChoice/1(FW_Data_Source), CmdTChoice/1(FW_Data_Source), CmdModeChoice/1(FW_Data_Source)
  Demux/3 -> CmdModeChoice/2(FW_CmdMode)
  CmdModeChoice/1(FW_Cmd_Mode) -> Cmd_Mode/1

== system GS_model/Subsystem2/EquipmentCmd/Fw1/Subsystem7/Subsystem3/Triggered Subsystem1 ==
  In1 : Inport
  Enable : EnablePort
  Out1 : Outport  InitialOutput=0
  wires:
  In1/1 -> Out1/1

== system GS_model/Subsystem2/EquipmentCmd/Fw1/Subsystem7/Subsystem4/FWDataSourceChoice ==
  note: 1 -- FW_Spd_422
      | 2 -- FW_Spd_UDP
      | 3 -- FW_Spd_FC
      |
      | 4 -- FW_T_422
      | 5 -- FW_T_UDP
      | 6 -- FW_T_FC
      |
      | 7 -- FW_Mode_422
      | 8 -- FW_Mode_UDP
      | 9 -- FW_Mode_FC
  FW_Data_Source : Inport
  FW_Cmd : Inport  Port=2
  CmdModeChoice : Subsystem
  CmdSpdChoice : Subsystem
  CmdTChoice : Subsystem
  Demux : Demux  Outputs=[3;3;3]
  Cmd_Mode : Outport
  Cmd_Spd : Outport  Port=2
  Cmd_T : Outport  Port=3
  wires:
  CmdModeChoice/1(FW_Cmd_Mode) -> Cmd_Mode/1
  Demux/3 -> CmdModeChoice/2(FW_CmdMode)
  FW_Data_Source/1 -> CmdModeChoice/1(FW_Data_Source), CmdTChoice/1(FW_Data_Source), CmdSpdChoice/1(FW_Data_Source)
  CmdSpdChoice/1(FW_Cmd_Spd) -> Cmd_Spd/1
  CmdTChoice/1(FW_Cmd_T) -> Cmd_T/1
  Demux/2 -> CmdTChoice/2(FW_CmdTorque)
  Demux/1 -> CmdSpdChoice/2(FW_CmdSpd)
  FW_Cmd/1 -> Demux/1

== system GS_model/Subsystem2/EquipmentCmd/Fw1/Subsystem7/Subsystem4/Triggered Subsystem1 ==
  In1 : Inport
  Enable : EnablePort
  Out1 : Outport  InitialOutput=0
  wires:
  In1/1 -> Out1/1

== system GS_model/Subsystem2/EquipmentCmd/Fw1/Subsystem7/Subsystem5/FWDataSourceChoice ==
  note: 1 -- FW_Spd_422
      | 2 -- FW_Spd_UDP
      | 3 -- FW_Spd_FC
      |
      | 4 -- FW_T_422
      | 5 -- FW_T_UDP
      | 6 -- FW_T_FC
      |
      | 7 -- FW_Mode_422
      | 8 -- FW_Mode_UDP
      | 9 -- FW_Mode_FC
  FW_Data_Source : Inport
  FW_Cmd : Inport  Port=2
  CmdModeChoice : Subsystem
  CmdSpdChoice : Subsystem
  CmdTChoice : Subsystem
  Demux : Demux  Outputs=[3;3;3]
  Cmd_Mode : Outport
  Cmd_Spd : Outport  Port=2
  Cmd_T : Outport  Port=3
  wires:
  FW_Cmd/1 -> Demux/1
  Demux/1 -> CmdSpdChoice/2(FW_CmdSpd)
  Demux/2 -> CmdTChoice/2(FW_CmdTorque)
  CmdTChoice/1(FW_Cmd_T) -> Cmd_T/1
  CmdSpdChoice/1(FW_Cmd_Spd) -> Cmd_Spd/1
  FW_Data_Source/1 -> CmdSpdChoice/1(FW_Data_Source), CmdTChoice/1(FW_Data_Source), CmdModeChoice/1(FW_Data_Source)
  Demux/3 -> CmdModeChoice/2(FW_CmdMode)
  CmdModeChoice/1(FW_Cmd_Mode) -> Cmd_Mode/1

== system GS_model/Subsystem2/EquipmentCmd/Fw1/Subsystem7/Subsystem5/Triggered Subsystem1 ==
  In1 : Inport
  Enable : EnablePort
  Out1 : Outport  InitialOutput=0
  wires:
  In1/1 -> Out1/1

== system GS_model/Subsystem2/EquipmentCmd/Fw1/Subsystem7/Subsystem6/FWDataSourceChoice ==
  note: 1 -- FW_Spd_422
      | 2 -- FW_Spd_UDP
      | 3 -- FW_Spd_FC
      |
      | 4 -- FW_T_422
      | 5 -- FW_T_UDP
      | 6 -- FW_T_FC
      |
      | 7 -- FW_Mode_422
      | 8 -- FW_Mode_UDP
      | 9 -- FW_Mode_FC
  FW_Data_Source : Inport
  FW_Cmd : Inport  Port=2
  CmdModeChoice : Subsystem
  CmdSpdChoice : Subsystem
  CmdTChoice : Subsystem
  Demux : Demux  Outputs=[3;3;3]
  Cmd_Mode : Outport
  Cmd_Spd : Outport  Port=2
  Cmd_T : Outport  Port=3
  wires:
  CmdModeChoice/1(FW_Cmd_Mode) -> Cmd_Mode/1
  Demux/3 -> CmdModeChoice/2(FW_CmdMode)
  FW_Data_Source/1 -> CmdModeChoice/1(FW_Data_Source), CmdTChoice/1(FW_Data_Source), CmdSpdChoice/1(FW_Data_Source)
  CmdSpdChoice/1(FW_Cmd_Spd) -> Cmd_Spd/1
  CmdTChoice/1(FW_Cmd_T) -> Cmd_T/1
  Demux/2 -> CmdTChoice/2(FW_CmdTorque)
  Demux/1 -> CmdSpdChoice/2(FW_CmdSpd)
  FW_Cmd/1 -> Demux/1

== system GS_model/Subsystem2/EquipmentCmd/Fw1/Subsystem7/Subsystem6/Triggered Subsystem1 ==
  In1 : Inport
  Enable : EnablePort
  Out1 : Outport  InitialOutput=0
  wires:
  In1/1 -> Out1/1

== system GS_model/Subsystem2/Subsystem/Actuator/Engine/Subsystem/Engine ==
  FireSwitch : Inport
  FireTime : Inport  Port=2
  Eg_PrepareTime : Inport  Port=3
  Eg_r_L_L : Inport  Port=4
  Cent : Inport  Port=5
  Eg_Dir : Inport  Port=6
  Eg_F : Inport  Port=7
  Eg_Fire_Pause : Inport  Port=8
  3x3 Cross Product : sharedutil/3x3 Cross Product  aMode=aMode
      settings: SourceProductBaseCode=AE,PW,MT,VE,VP
  Compare To Zero : simulink/Logic and Bit Operations/Compare To Zero  relop===  OutDataTypeStr=boolean
  Compare To Zero1 : simulink/Logic and Bit Operations/Compare To Zero  relop===  OutDataTypeStr=boolean
  Constant : Constant
  Data Type Conversion{,1..4} (5 alike) : DataTypeConversion
  Demux5 : Demux  Outputs=[1;1]
  Discrete-Time Integrator : DiscreteIntegrator  ExternalReset=level  SampleTime=T_Simu  ICPrevOutput=DiscIntNeverNeededParam  ICPrevScaledInput=DiscIntNeverNeededParam
  Discrete-Time Integrator1 : DiscreteIntegrator  ExternalReset=level  SampleTime=T_Simu  ICPrevOutput=DiscIntNeverNeededParam  ICPrevScaledInput=DiscIntNeverNeededParam
  Discrete-Time Integrator2 : DiscreteIntegrator  ExternalReset=level  SampleTime=T_Simu  ICPrevOutput=DiscIntNeverNeededParam  ICPrevScaledInput=DiscIntNeverNeededParam
  Logical Operator1 : Logic  Operator=OR  AllPortsSameDT=off  OutDataTypeStr=boolean
  Product : Product
  Product1 : Product  Inputs=4  SaturateOnIntegerOverflow=on  OutDataTypeStr=Inherit: Same as first input
  Product3 : Product  SaturateOnIntegerOverflow=on  OutDataTypeStr=Inherit: Same as first input
  Relational Operator : RelationalOperator  Operator=>  OutDataTypeStr=boolean  RndMeth=Simplest
  Relational Operator2 : RelationalOperator  Operator=<=  OutDataTypeStr=boolean  RndMeth=Simplest
  Relational Operator3 : RelationalOperator  Operator=>  OutDataTypeStr=boolean  RndMeth=Simplest
  Sum : Sum  Inputs=-+|
  T_Engine : Outport
  F_EP : Outport  Port=2
  wires:
  Eg_Dir/1 -> Product3/1
  FireSwitch/1 -> Compare To Zero/1, Discrete-Time Integrator/1
  Product1/1 -> Product3/2
  Compare To Zero/1 -> Data Type Conversion/1
  Product3/1 -> F_EP/1, 3x3 Cross Product/2
  Discrete-Time Integrator/1 -> Relational Operator/1
  Eg_F/1 -> Product1/1
  Relational Operator/1 -> Data Type Conversion1/1
  Data Type Conversion/1 -> Discrete-Time Integrator1/2, Discrete-Time Integrator/2
  Sum/1 -> 3x3 Cross Product/1
  Cent/1 -> Sum/1
  3x3 Cross Product/1 -> T_Engine/1
  Eg_r_L_L/1 -> Sum/2
  Eg_PrepareTime/1 -> Relational Operator/2
  Discrete-Time Integrator1/1 -> Relational Operator2/1
  Relational Operator2/1 -> Data Type Conversion2/1
  FireTime/1 -> Relational Operator2/2
  Demux5/1 -> Compare To Zero1/1
  Compare To Zero1/1 -> Logical Operator1/1, Data Type Conversion3/1
  Data Type Conversion3/1 -> Discrete-Time Integrator2/2
  Constant/1 -> Discrete-Time Integrator2/1
  Demux5/2 -> Relational Operator3/2
  Discrete-Time Integrator2/1 -> Relational Operator3/1
  Relational Operator3/1 -> Logical Operator1/2
  Data Type Conversion4/1 -> Product/1, Product1/2
  Logical Operator1/1 -> Data Type Conversion4/1
  Data Type Conversion2/1 -> Product1/4
  Data Type Conversion1/1 -> Product/2, Product1/3
  Product/1 -> Discrete-Time Integrator1/1
  Eg_Fire_Pause/1 -> Demux5/1

== system GS_model/Subsystem2/Subsystem/Actuator/Engine/Subsystem/Subsystem ==
  note: Dir_Choice/Switch/X/Y/Z
  Eg_Dir0 : Inport
  Eg_Dir_Set : Inport  Port=2
  Num : Inport  Port=3
  Compare To Constant : simulink/Logic and Bit Operations/Compare To Constant  relop===  const=0  OutDataTypeStr=boolean
  Demux : Demux  Outputs=[1;4]
  Demux5 : Demux  Outputs=[1;3]
  Logical Operator : Logic  Operator=OR  AllPortsSameDT=off  OutDataTypeStr=boolean
  Normalize Vector : vrlib/Utilities/Normalize Vector  maxzero=0
  Relational Operator1 : RelationalOperator  Operator===  OutDataTypeStr=boolean  RndMeth=Simplest
  Switch : Switch  Criteria=u2 > Threshold
  Triggered Subsystem1 : Subsystem  TreatAsAtomicUnit=on
      mask Display: disp('FWChoice')
  Eg_Dir : Outport
  wires:
  Demux/1 -> Relational Operator1/2, Compare To Constant/1
  Demux5/2 -> Switch/1
  Num/1 -> Relational Operator1/1
  Triggered Subsystem1/1(Out1) -> Demux5/1
  Logical Operator/1 -> Triggered Subsystem1/Enable
  Switch/1 -> Normalize Vector/1
  Demux/2 -> Triggered Subsystem1/1(In1)
  Eg_Dir0/1 -> Switch/3
  Demux5/1 -> Switch/2
  Eg_Dir_Set/1 -> Demux/1
  Compare To Constant/1 -> Logical Operator/2
  Relational Operator1/1 -> Logical Operator/1
  Normalize Vector/1 -> Eg_Dir/1

== system GS_model/Subsystem2/Subsystem/Actuator/Engine/Subsystem/Subsystem1 ==
  note: F_Choice/Switch/Value
  Eg_F0 : Inport
  Eg_F_Set : Inport  Port=2
  Num : Inport  Port=3
  Compare To Constant : simulink/Logic and Bit Operations/Compare To Constant  relop===  const=0  OutDataTypeStr=boolean
  Demux : Demux  Outputs=[1;2]
  Demux5 : Demux  Outputs=[1;1]
  Logical Operator : Logic  Operator=OR  AllPortsSameDT=off  OutDataTypeStr=boolean
  Relational Operator1 : RelationalOperator  Operator===  OutDataTypeStr=boolean  RndMeth=Simplest
  Switch : Switch  Criteria=u2 > Threshold
  Triggered Subsystem1 : Subsystem  TreatAsAtomicUnit=on
      mask Display: disp('FWChoice')
  Eg_F : Outport
  wires:
  Relational Operator1/1 -> Logical Operator/1
  Compare To Constant/1 -> Logical Operator/2
  Eg_F_Set/1 -> Demux/1
  Demux5/1 -> Switch/2
  Eg_F0/1 -> Switch/3
  Demux/2 -> Triggered Subsystem1/1(In1)
  Switch/1 -> Eg_F/1
  Logical Operator/1 -> Triggered Subsystem1/Enable
  Triggered Subsystem1/1(Out1) -> Demux5/1
  Num/1 -> Relational Operator1/1
  Demux5/2 -> Switch/1
  Demux/1 -> Compare To Constant/1, Relational Operator1/2

== system GS_model/Subsystem2/Subsystem/Actuator/Engine/Subsystem/Subsystem2 ==
  note: FirePause_Choice/Switch/Value
  Eg_F_Set : Inport
  Num : Inport  Port=2
  Compare To Constant : simulink/Logic and Bit Operations/Compare To Constant  relop===  const=0  OutDataTypeStr=boolean
  Demux : Demux  Outputs=[1;2]
  Logical Operator : Logic  Operator=OR  AllPortsSameDT=off  OutDataTypeStr=boolean
  Relational Operator1 : RelationalOperator  Operator===  OutDataTypeStr=boolean  RndMeth=Simplest
  Triggered Subsystem1 : Subsystem  TreatAsAtomicUnit=on
      mask Display: disp('FWChoice')
  Eg_FirePause : Outport
  wires:
  Demux/1 -> Relational Operator1/2, Compare To Constant/1
  Num/1 -> Relational Operator1/1
  Triggered Subsystem1/1(Out1) -> Eg_FirePause/1
  Logical Operator/1 -> Triggered Subsystem1/Enable
  Demux/2 -> Triggered Subsystem1/1(In1)
  Eg_F_Set/1 -> Demux/1
  Compare To Constant/1 -> Logical Operator/2
  Relational Operator1/1 -> Logical Operator/1

== system GS_model/Subsystem2/Subsystem/Actuator/Engine/Subsystem1/Engine ==
  FireSwitch : Inport
  FireTime : Inport  Port=2
  Eg_PrepareTime : Inport  Port=3
  Eg_r_L_L : Inport  Port=4
  Cent : Inport  Port=5
  Eg_Dir : Inport  Port=6
  Eg_F : Inport  Port=7
  Eg_Fire_Pause : Inport  Port=8
  3x3 Cross Product : sharedutil/3x3 Cross Product  aMode=aMode
      settings: SourceProductBaseCode=AE,PW,MT,VE,VP
  Compare To Zero : simulink/Logic and Bit Operations/Compare To Zero  relop===  OutDataTypeStr=boolean
  Compare To Zero1 : simulink/Logic and Bit Operations/Compare To Zero  relop===  OutDataTypeStr=boolean
  Constant : Constant
  Data Type Conversion{,1..4} (5 alike) : DataTypeConversion
  Demux5 : Demux  Outputs=[1;1]
  Discrete-Time Integrator : DiscreteIntegrator  ExternalReset=level  SampleTime=T_Simu  ICPrevOutput=DiscIntNeverNeededParam  ICPrevScaledInput=DiscIntNeverNeededParam
  Discrete-Time Integrator1 : DiscreteIntegrator  ExternalReset=level  SampleTime=T_Simu  ICPrevOutput=DiscIntNeverNeededParam  ICPrevScaledInput=DiscIntNeverNeededParam
  Discrete-Time Integrator2 : DiscreteIntegrator  ExternalReset=level  SampleTime=T_Simu  ICPrevOutput=DiscIntNeverNeededParam  ICPrevScaledInput=DiscIntNeverNeededParam
  Logical Operator1 : Logic  Operator=OR  AllPortsSameDT=off  OutDataTypeStr=boolean
  Product : Product
  Product1 : Product  Inputs=4  SaturateOnIntegerOverflow=on  OutDataTypeStr=Inherit: Same as first input
  Product3 : Product  SaturateOnIntegerOverflow=on  OutDataTypeStr=Inherit: Same as first input
  Relational Operator : RelationalOperator  Operator=>  OutDataTypeStr=boolean  RndMeth=Simplest
  Relational Operator2 : RelationalOperator  Operator=<=  OutDataTypeStr=boolean  RndMeth=Simplest
  Relational Operator3 : RelationalOperator  Operator=>  OutDataTypeStr=boolean  RndMeth=Simplest
  Sum : Sum  Inputs=-+|
  T_Engine : Outport
  F_EP : Outport  Port=2
  wires:
  Eg_Fire_Pause/1 -> Demux5/1
  Product/1 -> Discrete-Time Integrator1/1
  Data Type Conversion1/1 -> Product1/3, Product/2
  Data Type Conversion2/1 -> Product1/4
  Logical Operator1/1 -> Data Type Conversion4/1
  Data Type Conversion4/1 -> Product1/2, Product/1
  Relational Operator3/1 -> Logical Operator1/2
  Discrete-Time Integrator2/1 -> Relational Operator3/1
  Demux5/2 -> Relational Operator3/2
  Constant/1 -> Discrete-Time Integrator2/1
  Data Type Conversion3/1 -> Discrete-Time Integrator2/2
  Compare To Zero1/1 -> Data Type Conversion3/1, Logical Operator1/1
  Demux5/1 -> Compare To Zero1/1
  FireTime/1 -> Relational Operator2/2
  Relational Operator2/1 -> Data Type Conversion2/1
  Discrete-Time Integrator1/1 -> Relational Operator2/1
  Eg_PrepareTime/1 -> Relational Operator/2
  Eg_r_L_L/1 -> Sum/2
  3x3 Cross Product/1 -> T_Engine/1
  Cent/1 -> Sum/1
  Sum/1 -> 3x3 Cross Product/1
  Data Type Conversion/1 -> Discrete-Time Integrator/2, Discrete-Time Integrator1/2
  Relational Operator/1 -> Data Type Conversion1/1
  Eg_F/1 -> Product1/1
  Discrete-Time Integrator/1 -> Relational Operator/1
  Product3/1 -> 3x3 Cross Product/2, F_EP/1
  Compare To Zero/1 -> Data Type Conversion/1
  Product1/1 -> Product3/2
  FireSwitch/1 -> Discrete-Time Integrator/1, Compare To Zero/1
  Eg_Dir/1 -> Product3/1
